simulink model "canyongenerator"  (Simulink 7.2)
settings: Solver=ode45  StartTime=0.0  StopTime=10.0  RelTol=1e-3
settings Model: Creator=tlombaerts  LastModifiedBy=jelle
settings DataIOCC: LimitDataPoints=off
settings OptimizationCC: InitFltsAndDblsToZero=on
settings DebuggingCC: SaveWithParameterizedLinksMsg=none  SignalResolutionControl=TryResolveAllWithWarning
settings GRTTargetCC: TargetFcnLib=ansi_tfl_tmw.mat

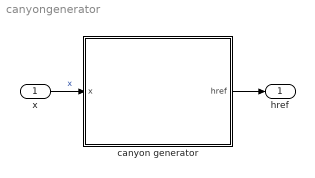
== system canyongenerator ==
  x : Inport  OutDataType=sfix(16)  OutScaling=2^0
  canyon generator : Subsystem
      mask Display: image(imread('refalt.jpg'))
  href : Outport  OutDataType=sfix(16)  OutScaling=2^0
  wires:
  x/1 -> canyon generator/1(x)  "x"
  canyon generator/1(href) -> href/1

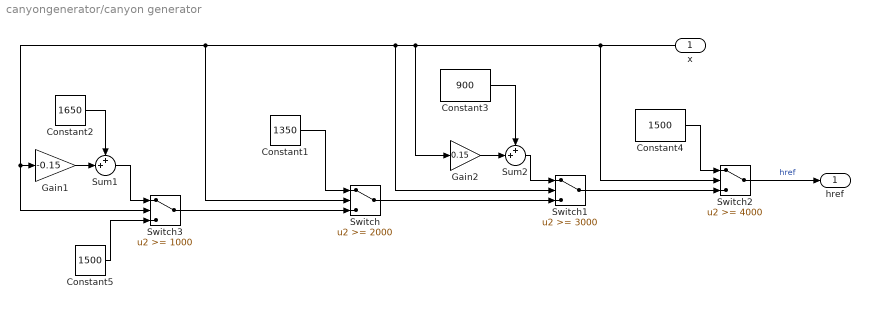
== system canyongenerator/canyon generator ==
  x : Inport  Orientation=left  OutDataType=sfix(16)  OutScaling=2^0
  Constant1 : Constant  Value=1350  OutDataType=sfix(16)  OutScaling=2^0
  Constant2 : Constant  Value=1650  OutDataType=sfix(16)  OutScaling=2^0
  Constant3 : Constant  Value=900  OutDataType=sfix(16)  OutScaling=2^0
  Constant4 : Constant  Value=1500  OutDataType=sfix(16)  OutScaling=2^0
  Constant5 : Constant  Value=1500  OutDataType=sfix(16)  OutScaling=2^0
  Gain1 : Gain  Gain=-0.15  ParameterDataType=sfix(16)  ParameterScaling=2^0  OutDataType=sfix(16)  OutScaling=2^0
  Gain2 : Gain  Gain=0.15  ParameterDataType=sfix(16)  ParameterScaling=2^0  OutDataType=sfix(16)  OutScaling=2^0
  Sum1 : Sum  Inputs=++|  OutDataType=sfix(16)  OutScaling=2^0
  Sum2 : Sum  Inputs=++|  OutDataType=sfix(16)  OutScaling=2^0
  Switch : Switch  Threshold=2000  ZeroCross=off
  Switch1 : Switch  Threshold=3000  ZeroCross=off
  Switch2 : Switch  Threshold=4000  ZeroCross=off
  Switch3 : Switch  Threshold=1000  ZeroCross=off
  href : Outport  OutDataType=sfix(16)  OutScaling=2^0
  wires:
  Constant1/1 -> Switch/1
  x/1 -> Switch2/2, Gain2/1, Switch1/2, Switch/2, Gain1/1, Switch3/2
  Switch/1 -> Switch1/3
  Gain2/1 -> Sum2/2
  Constant3/1 -> Sum2/1
  Sum2/1 -> Switch1/1
  Switch1/1 -> Switch2/3
  Constant4/1 -> Switch2/1
  Switch2/1 -> href/1  "href"
  Switch3/1 -> Switch/3
  Constant5/1 -> Switch3/3
  Sum1/1 -> Switch3/1
  Gain1/1 -> Sum1/2
  Constant2/1 -> Sum1/1
